simulink model "mintaveteles_PI_szabalyozo"  (Simulink 8.7)
settings: Solver=VariableStepAuto  StartTime=0.0  StopTime=T_sim  RelTol=1e-3
values from neighbouring files (symbols this model uses):
  K_C = 1/P1d.Numerator(2)*(1-exp(-Ts/T_cl))    [Sebessegszabalyozas_sim.m]
  P1d = c2d(sys,Ts,'zoh')    [Sebessegszabalyozas_sim.m]
  Ts = 0.1    [Sebessegszabalyozas_sim.m]
  z_d = -P1d.Denominator(2)    [Sebessegszabalyozas_sim.m]
settings Model: Creator=Mester Ádám  LastModifiedBy=Mester Ádám
settings DataIOCC: LimitDataPoints=off  SaveFormat=Dataset
settings DebuggingCC: UnderspecifiedInitializationDetection=Simplified  MergeDetectMultiDrivingBlocksExec=error
settings HardwareCC: ProdBitPerPointer=64  ProdLargestAtomicFloat=Float  ProdIntDivRoundTo=Zero  ProdEndianess=LittleEndian  ProdWordSize=64  ProdHWDeviceType=Intel->x86-64 (Windows64)
settings ModelReferenceCC: PropagateSignalLabelsOutOfModel=on
settings ConfigComp: CovModelRefEnable=off

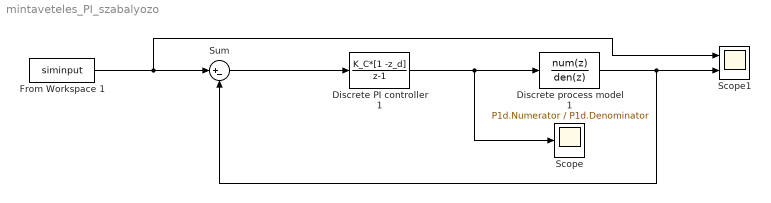
== system mintaveteles_PI_szabalyozo ==
  Discrete PI controller 1 : DiscreteTransferFcn  Numerator=K_C*[1 -z_d]  Denominator=[1 -1]  SampleTime=Ts
  Discrete process model 1 : DiscreteTransferFcn  Numerator=P1d.Numerator  Denominator=P1d.Denominator  SampleTime=Ts
  From Workspace 1 : FromWorkspace  VariableName=siminput  SampleTime=Ts
  Scope : Scope
  Scope1 : Scope  NumInputPorts=2
  Sum : Sum  Inputs=|+-
  wires:
  Discrete process model 1/1 -> Sum/2, Scope1/2
  From Workspace 1/1 -> Scope1/1, Sum/1
  Sum/1 -> Discrete PI controller 1/1
  Discrete PI controller 1/1 -> Scope/1, Discrete process model 1/1
